simulink model "ex2_2"  (R2020b)
settings: Solver=VariableStepAuto  StartTime=0.0  StopTime=10.0  RelTol=1e-3
values from neighbouring files (symbols this model uses):
  A = [0, 0, 1, 0; 0, 0, 0, 1; -6005, 5, -250, 250; 1, -1, 50, -50]    [ex2_2matlab.m]
  B = [0; 0; 6000; 0]    [ex2_2matlab.m]
  C = [1, 0, 0, 0; 0, 1, 0, 0]    [ex2_2matlab.m]
  D = [0; 0]    [ex2_2matlab.m]
  denominador_G1 = [2000, 600000, 12012000, 600000000, 12000000]    [ex2_2matlab.m]
  denominador_G2 = [2000, 600000, 12012000, 600000000, 12000000]    [ex2_2matlab.m]
  numerador_G1 = [12000000, 600000000, 12000000]    [ex2_2matlab.m]
  numerador_G2 = [600000000, 12000000]    [ex2_2matlab.m]
libraries: simulink x1
settings Model: Creator=artur  LastModifiedBy=artur

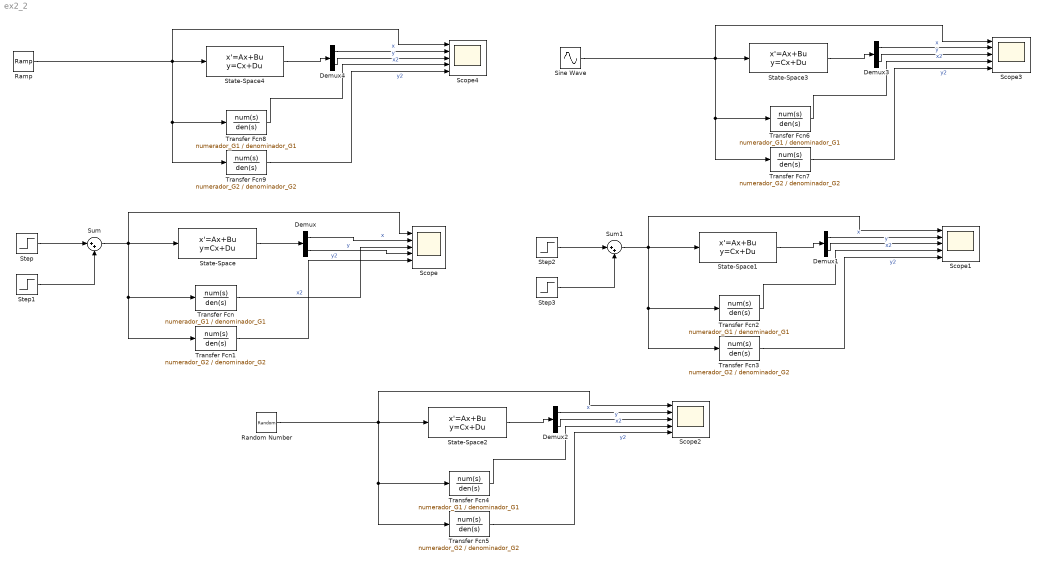
== system ex2_2 ==
  Demux{,1..4} (5 alike) : Demux  Outputs=2
  Ramp : simulink/Sources/Ramp  slope=1  start=4  InitialOutput=0
  Random Number : RandomNumber  SampleTime=0.1
  Scope{,1..4} (5 alike) : Scope  NumInputPorts=5
  Sine Wave : Sin  SampleTime=0
  State-Space{,1..4} (5 alike) : StateSpace  A=A  B=B  C=C  D=D  InitialCondition=0
  Step : Step  Time=3  SampleTime=0
  Step1 : Step  Time=4  After=-1  SampleTime=0
  Step2 : Step  Time=3  After=-1  SampleTime=0
  Step3 : Step  Time=4  SampleTime=0
  Sum : Sum  Inputs=|++
  Sum1 : Sum  Inputs=|++
  Transfer Fcn{,2,4,6,8} (5 alike) : TransferFcn  Numerator=numerador_G1  Denominator=denominador_G1
  Transfer Fcn{1,3,5,7,9} (5 alike) : TransferFcn  Numerator=numerador_G2  Denominator=denominador_G2
  wires:
  State-Space1/1 -> Demux1/1
  Transfer Fcn3/1 -> Scope1/5  "y2"
  Ramp/1 -> Transfer Fcn9/1, Transfer Fcn8/1, Scope4/1, State-Space4/1
  Demux/2 -> Scope/4  "y"
  Transfer Fcn9/1 -> Scope4/5  "y2"
  Sum1/1 -> Transfer Fcn2/1, Transfer Fcn3/1, Scope1/1, State-Space1/1
  State-Space2/1 -> Demux2/1
  Demux4/2 -> Scope4/3  "y"
  Transfer Fcn7/1 -> Scope3/5  "y2"
  State-Space4/1 -> Demux4/1
  Demux2/2 -> Scope2/3  "y"
  Step/1 -> Sum/1
  Sine Wave/1 -> Transfer Fcn7/1, Transfer Fcn6/1, Scope3/1, State-Space3/1
  Demux3/1 -> Scope3/2  "x"
  Demux4/1 -> Scope4/2  "x"
  Sum/1 -> Transfer Fcn1/1, Transfer Fcn/1, State-Space/1, Scope/1
  Demux/1 -> Scope/2  "x"
  Transfer Fcn4/1 -> Scope2/4  "x2"
  Demux3/2 -> Scope3/3  "y"
  Transfer Fcn5/1 -> Scope2/5  "y2"
  Transfer Fcn6/1 -> Scope3/4  "x2"
  Random Number/1 -> Transfer Fcn4/1, Transfer Fcn5/1, Scope2/1, State-Space2/1
  State-Space3/1 -> Demux3/1
  Transfer Fcn2/1 -> Scope1/4  "x2"
  Step3/1 -> Sum1/2
  Demux1/1 -> Scope1/2  "x"
  Transfer Fcn/1 -> Scope/3  "x2"
  Transfer Fcn1/1 -> Scope/5  "y2"
  Transfer Fcn8/1 -> Scope4/4  "x2"
  Demux1/2 -> Scope1/3  "y"
  Step2/1 -> Sum1/1
  Step1/1 -> Sum/2
  State-Space/1 -> Demux/1
  Demux2/1 -> Scope2/2  "x"
